simulink library "xbsIndex_r3"  (Simulink 6.1)
(part 3 of 4)

      | iCy=iHeight/2;
      | [logoX, logoY] = xlogo(iPos);
      | aw = 3;
      | ah = 7;
      | arrowX = [0 (-aw) (-aw) 0 0 (1) (1) (aw+1) (aw+1) (1)];
      | arrowY = [(ah-1) (ah-aw-1) (ah-aw) (ah) (-ah) (-ah) (ah) (ah-aw) (ah-aw-1) (ah-1)];
      | arrowX = arrowX + iCx - 1 - 3.5*length(str);
      | arrowY = arrowY + iCy + 3;
      | 
      | 
      | % one time added for param list
      | latancy = 0;
      | precision0 = 1;
      | dblOvrd = dbl_ovrd;
      | ratio = sample_ratio;
      | copySamples = copy_samples;
      | 
      | 
      | % just pass everything to s-function
      | sfcn_mwsv__ = get_param(gcb, 'MaskWSVariables');
      | 
      | nport = get_param(gcbh, 'ports');
      | nin = nport(1);
      | nout = nport(2);
      mask Help: eval('xlWeb(xlhtmldoclink(''Up Sample''))');
      mask Display:
      | patch([0 iWidth iWidth 0],[0 0 iHeight iHeight] , bg);
      | patch(logoX,logoY , fg);
      | plot(arrowX,arrowY);
      | disp(str);
      | 
      | ;plot([0 0 iWidth iWidth 0], [0 iHeight iHeight 0 0]);
  Viterbi Decoder : S-Function  FunctionName=xldeprecated  Parameters=nin,nout  mask(Xilinx Viterbi Decoder){clength=7, dual_decoding=off, conv_codes=[117 127], conv_codes2=[117 127], tb_length=36, coding=Soft, data_format=Signed Magnitude, puncturing=off, best_state=off, best_state_wr=0, red_latency=off, explicit_period=off, period=1, has_ber=off, ber_rate=20, has_norm=off, rst=off, en=off, dbl_ovrd=off, show_param=off, architecture=Parallel, optimization=Area, use_rpm=on, gen_core=off, xl_area=[0, 0, 0, 0, 0, 0, 0], xl_use_area=off}
      mask prompts: clength "Constraint Length"; dual_decoding "Use Dual Decoder"; conv_codes "Convolution Code Array 1 (octal)"; conv_codes2 "Convolution Code Array 2 (octal)"; tb_length "Traceback Length"; data_format "Data Format"; puncturing "Use External Puncturing"; best_state "Use Best State"; best_state_wr "Width Reduction"; red_latency "Reduce Latency"; explicit_period "Use Explicit Sample Period"; period "Sample Period  (use -1 to inherit first known input period)"; has_ber "Provide Bit Error Rate Port"; ber_rate "Number of Input Samples for Error Count"; has_norm "Provide Normalization Port"; rst "Provide Reset Port"; en "Provide Enable Port"; dbl_ovrd "Override with Doubles"; show_param "---------------------- Show Implementation Parameters -----------------------------------------------------------------------------------"; architecture "Architecture Type"; use_rpm "Use Placement Information for Core"; gen_core "Generate Core"; xl_area "FPGA Area [Slices, FFs, BRAMs, LUTs, IOBs, Emb. Mults, TBUFs]"; xl_use_area "Use Area Above For Estimation"
      mask help:
      | BLOCK IS OUT OF DATE.
      |
      | This block is from an outdated copy of the Xilinx Blockset. Please run xlUpdateModel('<model-name>') to update to the latest version.
      mask init:
      | xlmeta;
      | code_struct = xlconvertcodes(clength,conv_codes);
      | code_struct2 = xlconvertcodes(clength,conv_codes2);
      | output_rate = code_struct.output_rate;
      | output_rate2 = code_struct2.output_rate;
      | for i=1:output_rate,
      |   eval(sprintf('ccode%d = fliplr(code_struct.code%d);',i,i));
      | end
      | ccsucc = code_struct.success;
      | ccerror = code_struct.errorCode;
      | %find out the maximum rate
      | if(dual_decoding == 1)
      |   if(output_rate > output_rate2)
      | 	 max_output_rate = output_rate;
      |   else
      | 	 max_output_rate = output_rate2;
      |   end
      |   for i=1:output_rate2,
      |     eval(sprintf('ccode2_%d = fliplr(code_struct2.code%d);',i,i));
      |   end
      |   ccsucc2 = code_struct2.success;
      |   ccerror2 = code_struct2.errorCode;
      | else
      |   max_output_rate = output_rate;
      | end
      | num2 = 1; num3 = 1; num4 = 1; num5 = 1; 
      | num1 = 1;
      | num6 = 1; ostr6 = ''; num7 = 1; ostr7 = '';
      | ostr1 = '';
      | selPortNum = 1; biPortNum = 1;
      | ostr2 = ''; ostr3 = ''; ostr4 = ''; ostr5 = '';
      | selPortStr = ''; biPortStr = '';
      | boPort =2; boPortStr = 'vout';
      | rfdPortNum = 2; rfdPortStr = 'vout';
      | normPortNum = 2; normPortStr = 'vout';
      | berPortStr = 'vout'; berdonePortStr = 'vout';
      | berPortNum = 2; berdonePortNum = 2;
      | % setup default values for erase ports
      | for i = 1:7,
      |   eval(sprintf('erasePortStr%d = ''din1'';',i-1))
      |   eval(sprintf('erasePortNum%d = 1;',i-1))
      | end
      | nextPort = 2;
      | if(puncturing == 0) %no puncturing
      |  % set up input ports
      |   for j = 2:max_output_rate,
      |     eval(sprintf('ostr%d = ''din%d'';',j,j));
      |     eval(sprintf('num%d = %d;',j,j));
      |   end
      |   nextPort = max_output_rate + 1;
      | else %external puncturing
      |   for j = 1:max_output_rate,
      |     eval(sprintf('ostr%d = ''din%d'';',j,j));
      |     eval(sprintf('num%d = %d;',j,2*j-1)); 	
      |     eval(sprintf('erasePortStr%d = ''erase%d'';',j-1,j));
      |     eval(sprintf('erasePortNum%d = %d;',j-1,2*j));
      |   end
      |   nextPort = 2*max_output_rate + 1;
      | end
      | if(dual_decoding == 1)
      | 	selPortNum = nextPort;
      | 	selPortStr = 'sel';
      | 	nextPort = nextPort + 1;
      | end
      | nextOutPort = 3;
      | if(has_ber == 1)
      | 	berdonePortStr = 'ber_done';
      | 	berPortStr = 'ber';
      | 	berPortNum = 3;
      | 	berdonePortNum = 4;
      | 	nextOutPort = 5;
      | end
      | 
      | if(has_norm == 1)
      | 	normPortStr = 'norm';
      | 	if(has_ber == 1)
      | 	    normPortNum = 5;nextOutPort = 6;
      | 	else
      | 		normPortNum = 3;
      | 		nextOutPort = 4;
      | 	end
      | end
      | if(architecture == 2) %serial
      | 	rfdPortNum = nextOutPort;
      | 	rfdPortStr = 'rfd';
      | end
      | vin_pin = nextPort;
      | nextPort = nextPort + 1;
      | [enPortNum,enPortStr,rstPortNum,rstPortStr] = xlport_en_rst(en,rst,nextPort);
      | [designRoot, family, part, speed, package, simulinkPeriod, sysclkPeriod, dbl_ovrd, trimVbit] = xlSysgenSettings(gcb,1,0);
      | trimVbit=1;
      | [bg,fg] = xlcmap_r3('PayCore',dbl_ovrd);
      | iPos = get_param(gcb,'Position');
      | iWidth=iPos(3)-iPos(1);
      | iHeight=iPos(4)-iPos(2);
      | iCx=iWidth/2;
      | iCy=iHeight/2;
      | [logoX, logoY] = xlogo(iPos);
      | 
      | % one time added for param list
      | hasRST = rst;
      | hasEN = en;
      | latency = 1;
      | dblOvrd = dbl_ovrd;
      | useCore = 1;
      | precision0 = 1;
      | precision1 = 1;
      | precision2 = 1;
      | precision3 = 1;
      | precision4 = 1;
      | precision5 = 1;
      | explicitClk = explicit_period;
      | rpm = use_rpm;
      | gen_core = 1;
      | 
      | dll_name= ['xlviterbi_v3_0_' int2str(clength) '.dll'];
      | xlviterbi_dll=[ xlFindSysgenRoot '\bin\' dll_name ];
      | if isempty(which(xlviterbi_dll)) == 1
      | 	orig_dll = which('xlviterbi_v3_0.dll');
      | 	copyfile(orig_dll,xlviterbi_dll);
      | end
      | 
      | % just pass everything to s-function
      | sfcn_mwsv__ = get_param(gcb, 'MaskWSVariables');
      | 
      | nport = get_param(gcbh, 'ports');
      | nin = nport(1);
      | nout = nport(2);
      mask Help: eval('xlWeb(xlhtmldoclink(''Viterbi Decoder''))');
      mask StyleString: edit,checkbox,edit,edit,edit,popup(Soft|Hard),popup(Signed Magnitude|Offset Binary),checkbox,checkbox,popup(0|1|2|3),checkbox,checkbox,edit,checkbox,edit,checkbox,checkbox,checkbox,checkbox,checkbox,popup(Parallel|Serial),popup(Area|Speed),checkbox,checkbox,edit,checkbox
      mask Display:
      | patch([0 iWidth iWidth 0],[0 0 iHeight iHeight] , bg);
      | patch(logoX,logoY , fg);
      | port_label('input',1,'din1');
      | port_label('input',num2,ostr2);
      | port_label('input',num3,ostr3);
      | port_label('input',num4,ostr4);
      | port_label('input',num5,ostr5);
      | port_label('input',num6,ostr6);
      | port_label('input',num7,ostr7);
      | port_label('input',erasePortNum0,erasePortStr0);
      | port_label('input',erasePortNum1,erasePortStr1);
      | port_label('input',erasePortNum2,erasePortStr2);
      | port_label('input',erasePortNum3,erasePortStr3);
      | port_label('input',erasePortNum4,erasePortStr4);
      | port_label('input',erasePortNum5,erasePortStr5);
      | port_label('input',erasePortNum6,erasePortStr6);
      | port_label('input',selPortNum,selPortStr);
      | port_label('input',vin_pin,'vin');
      | port_label('input',enPortNum,enPortStr);
      | port_label('input',rstPortNum,rstPortStr);
      | port_label('output',1,'dout' );
      | port_label('output',2,'vout');
      | port_label('output',rfdPortNum, rfdPortStr);
      | port_label('output',normPortNum,normPortStr);
      | port_label('output',berPortNum,berPortStr);
      | port_label('output',berdonePortNum,berdonePortStr);
      | plot([0 0 iWidth iWidth 0], [0 iHeight iHeight 0 0]);
